simulink subsystem "core"  (R2021b)
settings: Solver=VariableStepAuto  StartTime=0.0  StopTime=10.0  RelTol=1e-3
settings Model: Creator=Otonom  LastModifiedBy=Otonom

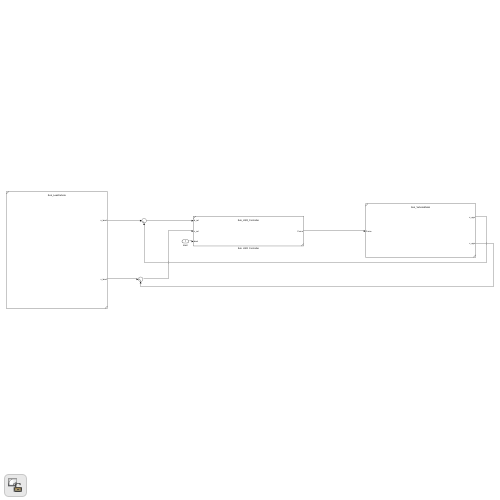
[thumbnail: Simulink's stored preview of the top-level diagram]
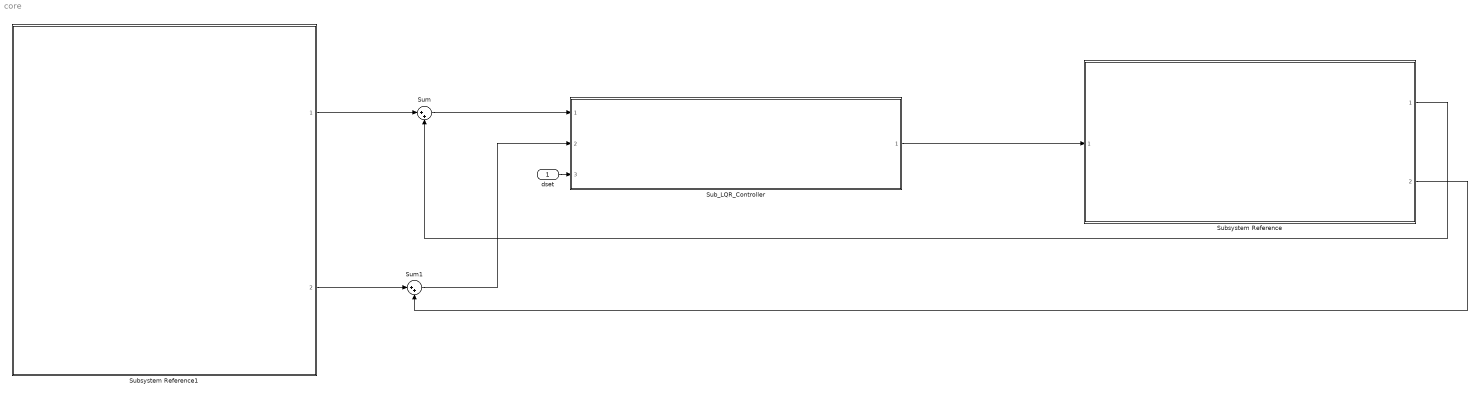
== system core ==
  dset : Inport
  Sub_LQR_Controller : Subsystem  ReferencedSubsystem=Sub_LQR_Controller
  Subsystem Reference : Subsystem  ReferencedSubsystem=Sub_VehicleModel
  Subsystem Reference1 : Subsystem  ReferencedSubsystem=Sub_LeadVehicle
  Sum : Sum  Inputs=|++
  Sum1 : Sum  Inputs=|++
  wires:
  dset/1 -> Sub_LQR_Controller/3
  Sum/1 -> Sub_LQR_Controller/1
  Subsystem Reference/1 -> Sum/2
  Sum1/1 -> Sub_LQR_Controller/2
  Subsystem Reference1/1 -> Sum/1
  Subsystem Reference/2 -> Sum1/2
  Sub_LQR_Controller/1 -> Subsystem Reference/1
  Subsystem Reference1/2 -> Sum1/1
